simulink model "ALG_Indication_Model"  (R2018b)
settings: configuration reference "FixedStepConfiguration" (kept outside this file)
libraries: simulink x8
settings Model: DataDictionary=DataDictionary.sldd  Creator=chris  LastModifiedBy=chris

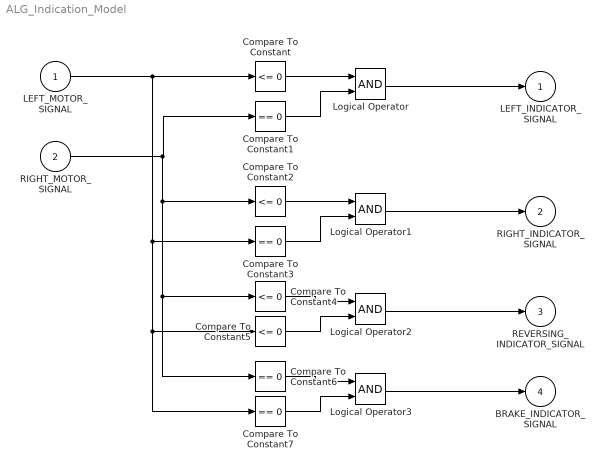
== system ALG_Indication_Model ==
  LEFT_MOTOR_SIGNAL : Inport
  RIGHT_MOTOR_SIGNAL : Inport  Port=2
  Compare To Constant{,2,4..5} (4 alike) : simulink/Logic and Bit Operations/Compare To Constant  relop=<=  const=0  OutDataTypeStr=boolean
  Compare To Constant{1,3,6..7} (4 alike) : simulink/Logic and Bit Operations/Compare To Constant  relop===  const=0  OutDataTypeStr=boolean
  Logical Operator{,1..3} (4 alike) : Logic  AllPortsSameDT=off  OutDataTypeStr=boolean
  LEFT_INDICATOR_SIGNAL : Outport
  RIGHT_INDICATOR_SIGNAL : Outport  Port=2
  REVERSING_INDICATOR_SIGNAL : Outport  Port=3
  BRAKE_INDICATOR_SIGNAL : Outport  Port=4
  wires:
  LEFT_MOTOR_SIGNAL/1 -> Compare To Constant7/1, Compare To Constant5/1, Compare To Constant3/1, Compare To Constant/1
  Compare To Constant/1 -> Logical Operator/1
  Compare To Constant1/1 -> Logical Operator/2
  RIGHT_MOTOR_SIGNAL/1 -> Compare To Constant6/1, Compare To Constant4/1, Compare To Constant2/1, Compare To Constant1/1
  Logical Operator/1 -> LEFT_INDICATOR_SIGNAL/1
  Logical Operator1/1 -> RIGHT_INDICATOR_SIGNAL/1
  Compare To Constant2/1 -> Logical Operator1/1
  Compare To Constant3/1 -> Logical Operator1/2
  Logical Operator2/1 -> REVERSING_INDICATOR_SIGNAL/1
  Compare To Constant4/1 -> Logical Operator2/1
  Compare To Constant5/1 -> Logical Operator2/2
  Compare To Constant7/1 -> Logical Operator3/2
  Compare To Constant6/1 -> Logical Operator3/1
  Logical Operator3/1 -> BRAKE_INDICATOR_SIGNAL/1
